simulink model "Bicycle_Model"  (R2017a)
settings: Solver=VariableStepAuto  StartTime=0.0  StopTime=inf  RelTol=1e-3
values from neighbouring files (symbols this model uses):
  A = 2.2    [model_params.m]
  Cd = 0.3    [model_params.m]
  Crr = 12.8    [model_params.m]
  Dm = 0.55    [model_params.m]
  Ktor = 1    [model_params.m]
  l = 4.564    [model_params.m]
  M = 1500    [model_params.m]
  n = 0.7    [model_params.m]
  Rho = 1.29    [model_params.m]
  Rw = 0.34    [model_params.m]
  Xd = 3.42    [model_params.m]
  Xg = 1.62    [model_params.m]
undefined symbols (not defined in the file or in its folder): magnitude
libraries: simulink x4
settings Model: Creator=DELL5521  LastModifiedBy=DELL5521

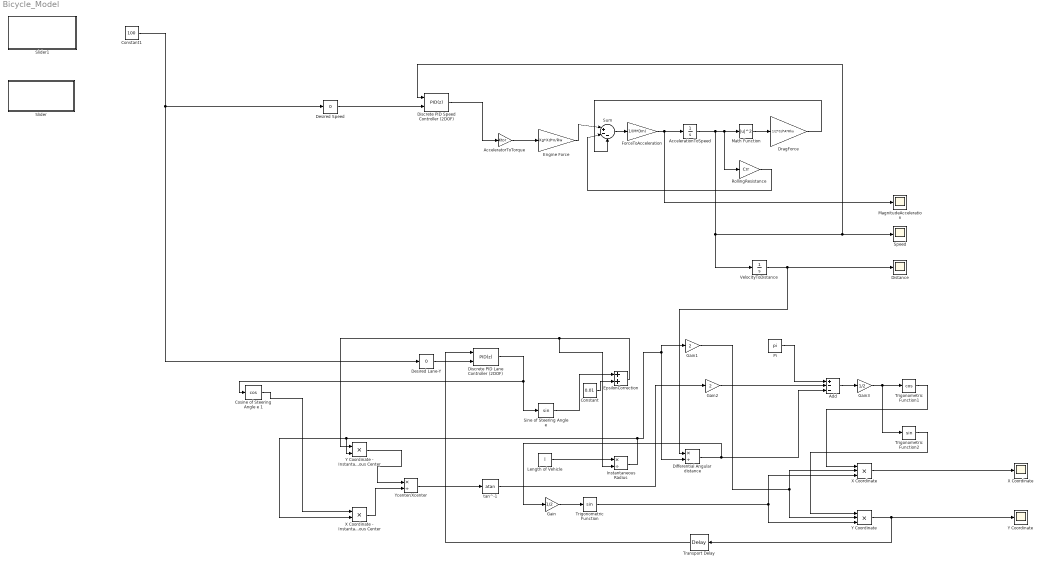
== system Bicycle_Model ==
  AccelerationToSpeed : Integrator
  AcceleratorToTorque : Gain  Gain=Ktor
  Add : Sum  Inputs=+--
  Constant : Constant  Value=0.01
  Constant1 : Constant  Value=100  VectorParams1D=off  OutMin=0  OutMax=100
  Cosine of Steering Angle e 1 : Trigonometry  Operator=cos
  Desired Lane-Y : simulink/Math Operations/Slider Gain  gain=0  low=0  high=1
  Desired Speed : simulink/Math Operations/Slider Gain  gain=0  low=0  high=1
  "Differential Angular distance " : Product  Inputs=*/
  Discrete PID Lane Controller (2DOF) : simulink/Continuous/PID Controller (2DOF)  Controller=PID  TimeDomain=Discrete-time  SampleTime=-1  IntegratorMethod=Forward Euler  FilterMethod=Forward Euler  Form=Parallel  UseFilter=on  ControllerParametersSource=internal  P=1  I=1  D=0  N=100  b=1  c=1  InitialConditionSource=internal  InitialConditionForIntegrator=0  InitialConditionForFilter=0  ExternalReset=none  LimitOutput=off  UpperSaturationLimit=inf  LowerSaturationLimit=-inf  LinearizeAsGain=off  AntiWindupMode=none  Kb=1  TrackingMode=off  Kt=1  PParamMin=[]  PParamMax=[]  IParamMin=[]  IParamMax=[]  DParamMin=[]  DParamMax=[]  NParamMin=[]  NParamMax=[]  bParamMin=[]  bParamMax=[]  cParamMin=[]  cParamMax=[]  KbParamMin=[]  KbParamMax=[]  KtParamMin=[]  KtParamMax=[]  POutMin=[]  POutMax=[]  IOutMin=[]  IOutMax=[]  DOutMin=[]  DOutMax=[]  NOutMin=[]  NOutMax=[]  bOutMin=[]  bOutMax=[]  cOutMin=[]  cOutMax=[]  KbOutMin=[]  KbOutMax=[]  KtOutMin=[]  KtOutMax=[]  IntegratorOutMin=[]  IntegratorOutMax=[]  FilterOutMin=[]  FilterOutMax=[]  SumOutMin=[]  SumOutMax=[]  Sum1OutMin=[]  Sum1OutMax=[]  Sum2OutMin=[]  Sum2OutMax=[]  Sum3OutMin=[]  Sum3OutMax=[]  SumI1OutMin=[]  SumI1OutMax=[]  SumI2OutMin=[]  SumI2OutMax=[]  SumI3OutMin=[]  SumI3OutMax=[]  SumDOutMin=[]  SumDOutMax=[]  SaturationOutMin=[]  SaturationOutMax=[]  IntegratorContinuousStateAttributes=''  IntegratorStateMustResolveToSignalObject=off  IntegratorRTWStateStorageClass=Auto  FilterContinuousStateAttributes=''  FilterStateMustResolveToSignalObject=off  FilterRTWStateStorageClass=Auto  DifferentiatorICPrevScaledInput=0  DifferentiatorOutMin=[]  DifferentiatorOutMax=[]  InitialConditionSetting=State (most efficient)
  Discrete PID Speed Controller (2DOF) : simulink/Continuous/PID Controller (2DOF)  Controller=PID  TimeDomain=Discrete-time  SampleTime=-1  IntegratorMethod=Forward Euler  FilterMethod=Forward Euler  Form=Parallel  UseFilter=on  ControllerParametersSource=internal  P=1  I=1  D=0  N=100  b=1  c=1  InitialConditionSource=internal  InitialConditionForIntegrator=0  InitialConditionForFilter=0  ExternalReset=none  LimitOutput=off  UpperSaturationLimit=inf  LowerSaturationLimit=-inf  LinearizeAsGain=off  AntiWindupMode=none  Kb=1  TrackingMode=off  Kt=1  PParamMin=[]  PParamMax=[]  IParamMin=[]  IParamMax=[]  DParamMin=[]  DParamMax=[]  NParamMin=[]  NParamMax=[]  bParamMin=[]  bParamMax=[]  cParamMin=[]  cParamMax=[]  KbParamMin=[]  KbParamMax=[]  KtParamMin=[]  KtParamMax=[]  POutMin=[]  POutMax=[]  IOutMin=[]  IOutMax=[]  DOutMin=[]  DOutMax=[]  NOutMin=[]  NOutMax=[]  bOutMin=[]  bOutMax=[]  cOutMin=[]  cOutMax=[]  KbOutMin=[]  KbOutMax=[]  KtOutMin=[]  KtOutMax=[]  IntegratorOutMin=[]  IntegratorOutMax=[]  FilterOutMin=[]  FilterOutMax=[]  SumOutMin=[]  SumOutMax=[]  Sum1OutMin=[]  Sum1OutMax=[]  Sum2OutMin=[]  Sum2OutMax=[]  Sum3OutMin=[]  Sum3OutMax=[]  SumI1OutMin=[]  SumI1OutMax=[]  SumI2OutMin=[]  SumI2OutMax=[]  SumI3OutMin=[]  SumI3OutMax=[]  SumDOutMin=[]  SumDOutMax=[]  SaturationOutMin=[]  SaturationOutMax=[]  IntegratorContinuousStateAttributes=''  IntegratorStateMustResolveToSignalObject=off  IntegratorRTWStateStorageClass=Auto  FilterContinuousStateAttributes=''  FilterStateMustResolveToSignalObject=off  FilterRTWStateStorageClass=Auto  DifferentiatorICPrevScaledInput=0  DifferentiatorOutMin=[]  DifferentiatorOutMax=[]  InitialConditionSetting=State (most efficient)
  Distance : Scope
  DragForce : Gain  Gain=1/2*Cd*A*Rho
  Engine Force : Gain  Gain=Xg*Xd*n/Rw
  EpsilonCorrection : Sum
  ForceToAcceleration : Gain  Gain=1/(M*Dm)
  Gain : Gain  Gain=1/2
  Gain1 : Gain  Gain=2
  Gain2 : Gain  Gain=2
  Gain3 : Gain  Gain=1/2
  "Instantaneous Radius " : Product  Inputs=*/
  Length of Vehicle : Constant  Value=l
  MagnitudeAcceleration : Scope
  Math Function : Math  Operator=magnitude^2  SaturateOnIntegerOverflow=on
  "Pi " : Constant  Value=pi
  RollingResistance : Gain  Gain=Crr
  "Sine of Steering Angle e " : Trigonometry
  Slider : Subsystem  DialogController=hmiCreateDDGDialog  IsWebBlock=on  mask(MWDashboardBlock){webBlockId=5041d8bd-c114-4b7e-8faf-3488bab7e256, webBlockType=slider, ShowInLibBrowser=on, ShowInitialText=on, HMISrcModelName=Bicycle_Model}
      mask prompts: webBlockId "WebBlock Id"; webBlockType "WebBlock Type"; HMISrcModelName "Source Model"
      mask help: SimulinkHMI:dialogs:SliderDialogDesc
      mask Help: helpview([docroot '/mapfiles/simulink.map'], 'hmi_slider')
      mask Display:
      | if strcmp(get_param(bdroot(gcb),'BlockDiagramType'), 'library')
      |     image([(matlabroot) '/toolbox/simulink/hmi/icons/Slider.png']);
      | end
  Slider1 : Subsystem  DialogController=hmiCreateDDGDialog  IsWebBlock=on  mask(MWDashboardBlock){webBlockId=c70cdcf2-7e67-4cc0-a498-f6269056a37b, webBlockType=slider, ShowInLibBrowser=on, ShowInitialText=on, HMISrcModelName=Bicycle_Model}
      mask prompts: webBlockId "WebBlock Id"; webBlockType "WebBlock Type"; HMISrcModelName "Source Model"
      mask help: SimulinkHMI:dialogs:SliderDialogDesc
      mask Help: helpview([docroot '/mapfiles/simulink.map'], 'hmi_slider')
      mask Display:
      | if strcmp(get_param(bdroot(gcb),'BlockDiagramType'), 'library')
      |     image([(matlabroot) '/toolbox/simulink/hmi/icons/Slider.png']);
      | end
  Speed : Scope
  Sum : Sum  Inputs=|+--
  Transport Delay : TransportDelay
  Trigonometric Function : Trigonometry
  Trigonometric Function1 : Trigonometry  Operator=cos
  Trigonometric Function2 : Trigonometry
  VelocityToDistance : Integrator
  X Coordinate : Scope
  "X Coordinate " : Product  Inputs=***
  X Coordinate - Instantaneous Center : Product  Inputs=**
  Y Coordinate : Scope
  "Y Coordinate " : Product  Inputs=***
  Y Coordinate - Instantaneous Center : Product  Inputs=**
  Ycenter/Xcenter : Product  Inputs=*/
  tan^-1 : Trigonometry  Operator=atan
  wires:
  Constant1/1 -> Desired Speed/1, Desired Lane-Y/1
  Engine Force/1 -> Sum/1
  Desired Speed/1 -> Discrete PID Speed Controller (2DOF)/2
  ForceToAcceleration/1 -> MagnitudeAcceleration/1, AccelerationToSpeed/1
  Sum/1 -> ForceToAcceleration/1
  Discrete PID Speed Controller (2DOF)/1 -> AcceleratorToTorque/1
  DragForce/1 -> Sum/3
  RollingResistance/1 -> Sum/2
  AcceleratorToTorque/1 -> Engine Force/1
  Math Function/1 -> DragForce/1
  AccelerationToSpeed/1 -> Discrete PID Speed Controller (2DOF)/1, Speed/1, VelocityToDistance/1, RollingResistance/1, Math Function/1
  VelocityToDistance/1 -> "Differential Angular distance "/1, Distance/1
  Length of Vehicle/1 -> "Instantaneous Radius "/1
  Ycenter/Xcenter/1 -> tan^-1/1
  Gain3/1 -> Trigonometric Function2/1, Trigonometric Function1/1
  Trigonometric Function2/1 -> "Y Coordinate "/1
  Add/1 -> Gain3/1
  Y Coordinate - Instantaneous Center/1 -> Ycenter/Xcenter/1
  "X Coordinate "/1 -> X Coordinate/1
  Trigonometric Function/1 -> "X Coordinate "/3, "Y Coordinate "/3
  tan^-1/1 -> Gain2/1
  Gain2/1 -> Add/2
  Discrete PID Lane Controller (2DOF)/1 -> "Sine of Steering Angle e "/1, Cosine of Steering Angle e 1/1
  Gain1/1 -> "X Coordinate "/2, "Y Coordinate "/2
  "Pi "/1 -> Add/1
  X Coordinate - Instantaneous Center/1 -> Ycenter/Xcenter/2
  "Instantaneous Radius "/1 -> X Coordinate - Instantaneous Center/2, Y Coordinate - Instantaneous Center/2, Gain1/1, "Differential Angular distance "/2
  "Sine of Steering Angle e "/1 -> EpsilonCorrection/1
  Cosine of Steering Angle e 1/1 -> X Coordinate - Instantaneous Center/1
  EpsilonCorrection/1 -> "Instantaneous Radius "/2, Y Coordinate - Instantaneous Center/1
  Trigonometric Function1/1 -> "X Coordinate "/1
  "Differential Angular distance "/1 -> Gain/1, Add/3
  Gain/1 -> Trigonometric Function/1
  Desired Lane-Y/1 -> Discrete PID Lane Controller (2DOF)/2
  Constant/1 -> EpsilonCorrection/2
  "Y Coordinate "/1 -> Transport Delay/1, Y Coordinate/1
  Transport Delay/1 -> Discrete PID Lane Controller (2DOF)/1

== system Bicycle_Model/Slider ==

== system Bicycle_Model/Slider1 ==
